simulink model "BatterySimulationCC"  (R2018b)
settings: Solver=VariableStepAuto  StartTime=0.0  StopTime=1  RelTol=1e-3
settings Model: Creator=GRosp  LastModifiedBy=GRosp

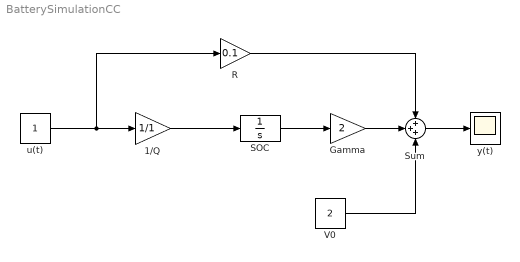
== system BatterySimulationCC ==
  1/Q : Gain  Gain=1/1
  "Gamma " : Gain  Gain=2
  R : Gain  Gain=0.1
  SOC : Integrator
  Sum : Sum  Inputs=+++
  V0 : Constant  Value=2
  u(t) : Constant
  "y(t) " : Scope
  wires:
  1/Q/1 -> SOC/1
  SOC/1 -> "Gamma "/1
  R/1 -> Sum/1
  "Gamma "/1 -> Sum/2
  V0/1 -> Sum/3
  Sum/1 -> "y(t) "/1
  u(t)/1 -> R/1, 1/Q/1
